simulink model "real_velocity_obs"  (R2023a)
settings: Solver=FixedStepAuto  StartTime=0.0  StopTime=20  FixedStep=0.0005  RelTol=1e-3
undefined symbols (not defined in the file): amp_disp, bias, c, c0, DiscIntNeverNeededParam, dT, freq_disp, k, k0, lsqr_method, m, m0
libraries: fl_lib x14, nesl_utility x8, simulink x3, sharedTrackingLibrary x2
settings Model: Creator=lucabeber  LastModifiedBy=robotics
settings OptimizationCC: ReuseModelBlockBuffer=off

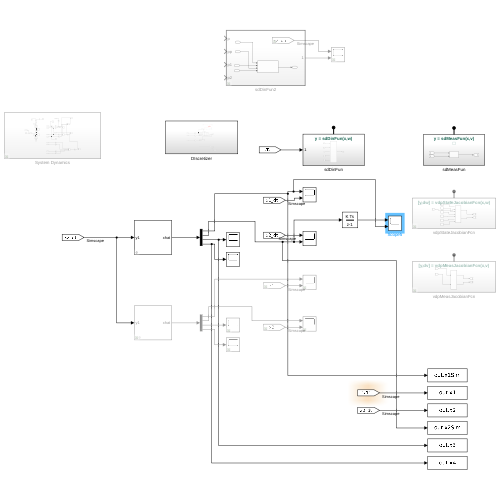
[thumbnail: Simulink's stored preview of the top-level diagram]
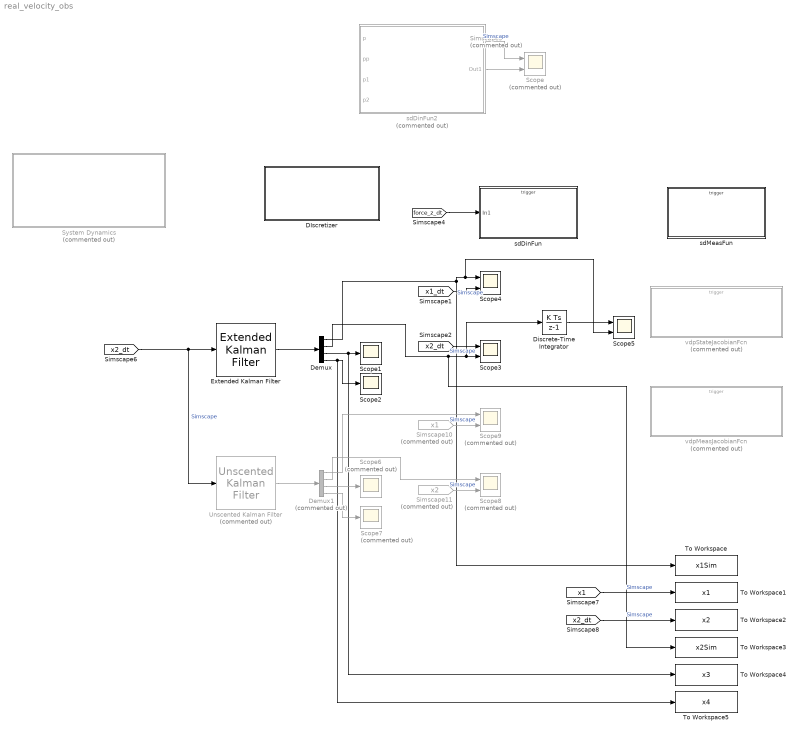
== system real_velocity_obs ==
  DIscretizer : Subsystem
  Demux : Demux
  Demux1 : Demux  Commented=on
  Discrete-Time Integrator : DiscreteIntegrator  SampleTime=-1  ICPrevOutput=DiscIntNeverNeededParam  ICPrevScaledInput=DiscIntNeverNeededParam
  Extended Kalman Filter : sharedTrackingLibrary/Extended Kalman Filter  StateTransitionFcn=sdDinFun  HasStateTransitionJacobianFcn=off  StateTransitionJacobianFcn=vdpStateJacobianFcn  HasAdditiveProcessNoise=Nonadditive  ProcessNoise=1e-5  HasTimeVaryingProcessNoise=off  HasStateTransitionFcnExtraArgument=0  InitialState=[0,0,1000,100]  InitialStateCovariance=[1,1,500,10]  MeasurementFcn1=sdMeasFun  HasMeasurementJacobianFcn1=off  MeasurementJacobianFcn1=vdpMeasJacobianFcn  HasMeasurementEnablePort1=off  HasAdditiveMeasurementNoise1=Nonadditive  MeasurementNoise1=0.000005  HasTimeVaryingMeasurementNoise1=off  HasMeasurementFcnExtraArgument1=0  HasMeasurementWrapping1=off  MeasurementFcn2=myMeasurementFcn  HasMeasurementJacobianFcn2=off  HasMeasurementEnablePort2=off  HasAdditiveMeasurementNoise2=Additive  MeasurementNoise2=1  HasTimeVaryingMeasurementNoise2=off  HasMeasurementFcnExtraArgument2=0  HasMeasurementWrapping2=off  MeasurementFcn3=myMeasurementFcn  HasMeasurementJacobianFcn3=off  HasMeasurementEnablePort3=off  HasAdditiveMeasurementNoise3=Additive  MeasurementNoise3=1  HasTimeVaryingMeasurementNoise3=off  HasMeasurementFcnExtraArgument3=0  HasMeasurementWrapping3=off  MeasurementFcn4=myMeasurementFcn  HasMeasurementJacobianFcn4=off  HasMeasurementEnablePort4=off  HasAdditiveMeasurementNoise4=Additive  MeasurementNoise4=1  HasTimeVaryingMeasurementNoise4=off  HasMeasurementFcnExtraArgument4=0  HasMeasurementWrapping4=off  MeasurementFcn5=myMeasurementFcn  HasMeasurementJacobianFcn5=off  HasMeasurementEnablePort5=off  HasAdditiveMeasurementNoise5=Additive  MeasurementNoise5=1  HasTimeVaryingMeasurementNoise5=off  HasMeasurementFcnExtraArgument5=0  HasMeasurementWrapping5=off  EnableMultirate=off  StateTransitionFcnSampleTime=1  MeasurementFcn1SampleTime=1  MeasurementFcn2SampleTime=1  MeasurementFcn3SampleTime=1  MeasurementFcn4SampleTime=1  MeasurementFcn5SampleTime=1  UseCurrentEstimator=on  OutputStateCovariance=off  DataType=double  SampleTime=dT  NumberOfMeasurements=1
  Scope : Scope  Commented=on  NumInputPorts=2
  Scope1 : Scope
  Scope2 : Scope
  Scope3 : Scope  NumInputPorts=2
  Scope4 : Scope  NumInputPorts=2
  Scope5 : Scope  NumInputPorts=2
  Scope6 : Scope  Commented=on
  Scope7 : Scope  Commented=on
  Scope8 : Scope  Commented=on  NumInputPorts=2
  Scope9 : Scope  Commented=on  NumInputPorts=2
  Simscape10 : From  Commented=on  GotoTag=x1  TagVisibility=global
  Simscape11 : From  Commented=on  GotoTag=x2  TagVisibility=global
  Simscape5 : From  Commented=on  GotoTag=x2_dot  TagVisibility=global
  System Dynamics : Subsystem  Commented=on
  To Workspace : ToWorkspace  VariableName=x1Sim  SampleTime=-1
  To Workspace1 : ToWorkspace  VariableName=x1  SampleTime=-1
  To Workspace2 : ToWorkspace  VariableName=x2  SampleTime=-1
  To Workspace3 : ToWorkspace  VariableName=x2Sim  SampleTime=-1
  To Workspace4 : ToWorkspace  VariableName=x3  SampleTime=-1
  To Workspace5 : ToWorkspace  VariableName=x4  SampleTime=-1
  Unscented Kalman Filter : sharedTrackingLibrary/Unscented Kalman Filter  Commented=on  StateTransitionFcn=sdDinFun  HasAdditiveProcessNoise=Nonadditive  ProcessNoise=0  HasTimeVaryingProcessNoise=off  HasStateTransitionFcnExtraArgument=0  InitialState=[0,0,0,0]  InitialStateCovariance=5000  Alpha=1e-3  Beta=2  Kappa=0  MeasurementFcn1=sdMeasFun  HasMeasurementEnablePort1=off  HasAdditiveMeasurementNoise1=Nonadditive  MeasurementNoise1=0.8  HasTimeVaryingMeasurementNoise1=off  HasMeasurementFcnExtraArgument1=0  HasMeasurementWrapping1=off  MeasurementFcn2=myMeasurementFcn  HasMeasurementEnablePort2=off  HasAdditiveMeasurementNoise2=Additive  MeasurementNoise2=1  HasTimeVaryingMeasurementNoise2=off  HasMeasurementFcnExtraArgument2=0  HasMeasurementWrapping2=off  MeasurementFcn3=myMeasurementFcn  HasMeasurementEnablePort3=off  HasAdditiveMeasurementNoise3=Additive  MeasurementNoise3=1  HasTimeVaryingMeasurementNoise3=off  HasMeasurementFcnExtraArgument3=0  HasMeasurementWrapping3=off  MeasurementFcn4=myMeasurementFcn  HasMeasurementEnablePort4=off  HasAdditiveMeasurementNoise4=Additive  MeasurementNoise4=1  HasTimeVaryingMeasurementNoise4=off  HasMeasurementFcnExtraArgument4=0  HasMeasurementWrapping4=off  MeasurementFcn5=myMeasurementFcn  HasMeasurementEnablePort5=off  HasAdditiveMeasurementNoise5=Additive  MeasurementNoise5=1  HasTimeVaryingMeasurementNoise5=off  HasMeasurementFcnExtraArgument5=0  HasMeasurementWrapping5=off  EnableMultirate=off  StateTransitionFcnSampleTime=1  MeasurementFcn1SampleTime=1  MeasurementFcn2SampleTime=1  MeasurementFcn3SampleTime=1  MeasurementFcn4SampleTime=1  MeasurementFcn5SampleTime=1  UseCurrentEstimator=on  OutputStateCovariance=off  DataType=double  SampleTime=dT  NumberOfMeasurements=1
      settings: LibrarySourceBlock=cstblocks/State Estimation/Unscented Kalman Filter
  sdDinFun : Subsystem  TreatAsAtomicUnit=on
  sdDinFun2 : Subsystem  Commented=on  TreatAsAtomicUnit=on
  sdMeasFun : Subsystem  TreatAsAtomicUnit=on
  vdpMeasJacobianFcn : Subsystem  Commented=on  TreatAsAtomicUnit=on
  vdpStateJacobianFcn : Subsystem  Commented=on  TreatAsAtomicUnit=on
  wires:
  sdDinFun2/1(Out1) -> Scope/2
  Simscape5/1 -> Scope/1  "Simscape"
  [x2_dt] -> Unscented Kalman Filter/1, Extended Kalman Filter/1  "Simscape"
  Extended Kalman Filter/1 -> Demux/1
  Demux/3 -> To Workspace4/1, Scope1/1
  Demux/4 -> To Workspace5/1, Scope2/1
  Demux/1 -> To Workspace/1, Scope5/2, Scope4/1
  Demux/2 -> To Workspace3/1, Discrete-Time Integrator/1, Scope3/2
  [x1_dt] -> Scope4/2  "Simscape"
  [force_z_dt] -> sdDinFun/1(In1)
  Demux1/4 -> Scope7/1
  Demux1/1 -> Scope9/1
  Demux1/3 -> Scope6/1
  Simscape11/1 -> Scope8/2  "Simscape"
  Unscented Kalman Filter/1 -> Demux1/1
  Demux1/2 -> Scope8/1
  Simscape10/1 -> Scope9/2  "Simscape"
  [x2_dt] -> Scope3/1  "Simscape"
  [x1] -> To Workspace1/1  "Simscape"
  [x2_dt] -> To Workspace2/1  "Simscape"
  Discrete-Time Integrator/1 -> Scope5/1

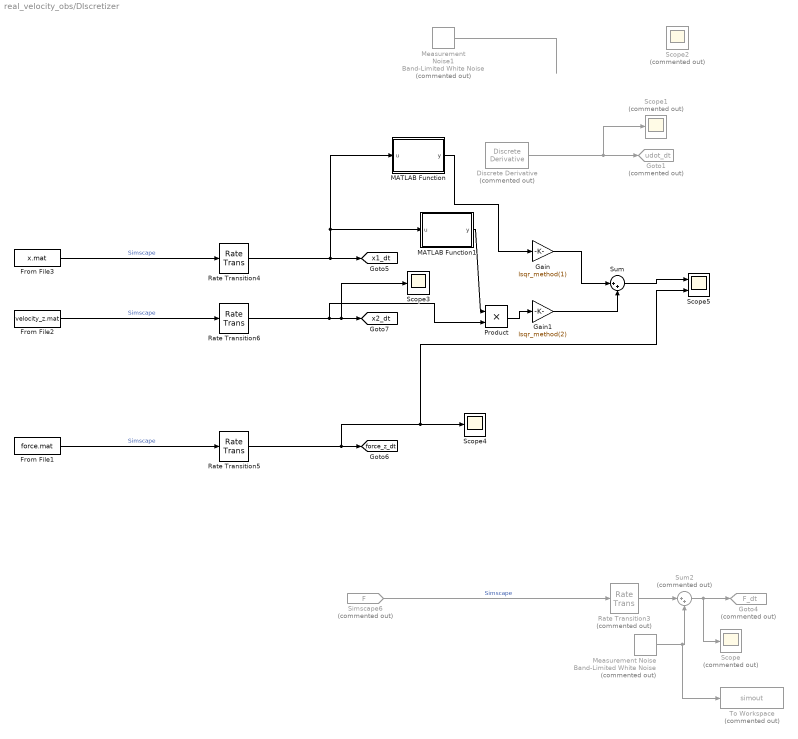
== system real_velocity_obs/DIscretizer ==
  Discrete Derivative : simulink/Discrete/Discrete Derivative  Commented=on  gainval=1.0  ICPrevScaledInput=0.0  OutMin=[]  OutMax=[]  OutDataType=fixdt(1, 16)  OutScaling=2^-10  DoSatur=off
  From File1 : FromFile  FileName=force.mat  SampleTime=dT
  From File2 : FromFile  FileName=velocity_z.mat  SampleTime=dT
  From File3 : FromFile  FileName=x.mat  SampleTime=dT
  Gain : Gain  Gain=lsqr_method(1)
  Gain1 : Gain  Gain=lsqr_method(2)
  Goto1 : Goto  Commented=on  GotoTag=udot_dt  TagVisibility=global
  Goto4 : Goto  Commented=on  GotoTag=F_dt  TagVisibility=global
  MATLAB Function : MATLAB Function  TreatAsAtomicUnit=on
  MATLAB Function1 : MATLAB Function  TreatAsAtomicUnit=on
  Measurement Noise : simulink/Sources/Band-Limited White Noise  Commented=on  Cov=4e-4  Ts=dT  seed=[23342]
  Measurement Noise1 : simulink/Sources/Band-Limited White Noise  Commented=on  Cov=0  Ts=dT  seed=[23342]
  Product : Product
  Rate Transition3 : RateTransition  Commented=on  OutPortSampleTime=dT
  Rate Transition4 : RateTransition  OutPortSampleTime=dT
  Rate Transition5 : RateTransition  OutPortSampleTime=dT
  Rate Transition6 : RateTransition  OutPortSampleTime=dT
  Scope : Scope  Commented=on
  Scope1 : Scope  Commented=on
  Scope2 : Scope  Commented=on
  Scope3 : Scope
  Scope4 : Scope
  Scope5 : Scope  NumInputPorts=2
  Simscape6 : From  Commented=on  GotoTag=F  TagVisibility=global
  Sum : Sum  Inputs=|++
  Sum2 : Sum  Commented=on  Inputs=|++
  To Workspace : ToWorkspace  Commented=on  VariableName=simout  SampleTime=-1
  tag scope: force_z_dt=global, x1_dt=global, x2_dt=global
  wires:
  Simscape6/1 -> Rate Transition3/1  "Simscape"
  Rate Transition3/1 -> Sum2/1
  Sum2/1 -> Scope/1, Goto4/1
  Measurement Noise/1 -> To Workspace/1, Sum2/2
  ? -> Discrete Derivative/1, Scope2/1
  Measurement Noise1/1 -> ?
  Discrete Derivative/1 -> Scope1/1, Goto1/1
  Rate Transition4/1 -> MATLAB Function1/1(u), MATLAB Function/1(u), [x1_dt]
  From File3/1 -> Rate Transition4/1  "Simscape"
  From File2/1 -> Rate Transition6/1  "Simscape"
  Rate Transition6/1 -> Product/2, Scope3/1, [x2_dt]
  From File1/1 -> Rate Transition5/1  "Simscape"
  Rate Transition5/1 -> Scope5/2, Scope4/1, [force_z_dt]
  Sum/1 -> Scope5/1
  Gain/1 -> Sum/1
  Gain1/1 -> Sum/2
  MATLAB Function/1(y) -> Gain/1
  Product/1 -> Gain1/1
  MATLAB Function1/1(y) -> Product/1

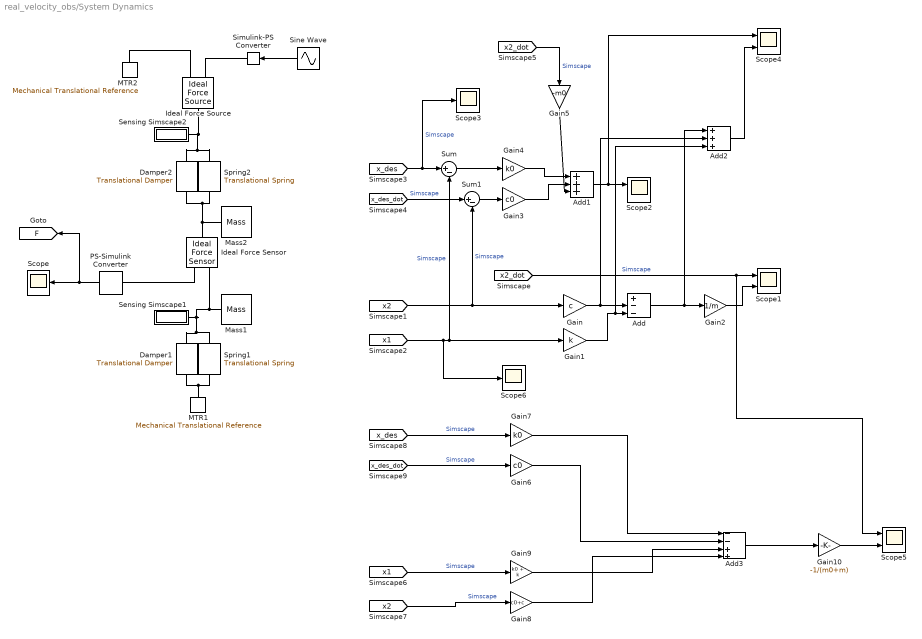
== system real_velocity_obs/System Dynamics ==
  " Spring1" : fl_lib/Mechanical/Translational Elements/Translational Spring  spr_rate=k N/m  v_specify=off  v_priority=None  v=0 m/s  v_nominal_specify=off  v_nominal_unit=m/s  v_nominal_value=1  f_specify=off  f_priority=None  f=0 N  f_nominal_specify=off  f_nominal_unit=N  f_nominal_value=1  x_specify=off  x_priority=High  x=0 m  x_nominal_specify=off  x_nominal_unit=m  x_nominal_value=1
  " Spring2" : fl_lib/Mechanical/Translational Elements/Translational Spring  spr_rate=k0 N/m  v_specify=off  v_priority=None  v=0 m/s  v_nominal_specify=off  v_nominal_unit=m/s  v_nominal_value=1  f_specify=off  f_priority=None  f=0 N  f_nominal_specify=off  f_nominal_unit=N  f_nominal_value=1  x_specify=off  x_priority=High  x=0 m  x_nominal_specify=off  x_nominal_unit=m  x_nominal_value=1
  Add : Sum  Inputs=+--
  Add1 : Sum  Inputs=+++
  Add2 : Sum  Inputs=+++
  Add3 : Sum  Inputs=--++
  Damper1 : fl_lib/Mechanical/Translational Elements/Translational Damper  D=c N/(m/s)  v_specify=off  v_priority=High  v=0 m/s  v_nominal_specify=off  v_nominal_unit=m/s  v_nominal_value=1  f_specify=off  f_priority=High  f=0 N  f_nominal_specify=off  f_nominal_unit=N  f_nominal_value=1
  Damper2 : fl_lib/Mechanical/Translational Elements/Translational Damper  D=c0 N/(m/s)  v_specify=off  v_priority=High  v=0 m/s  v_nominal_specify=off  v_nominal_unit=m/s  v_nominal_value=1  f_specify=off  f_priority=High  f=0 N  f_nominal_specify=off  f_nominal_unit=N  f_nominal_value=1
  Gain : Gain  Gain=c
  Gain1 : Gain  Gain=k
  Gain10 : Gain  Gain=-1/(m0+m)
  Gain2 : Gain  Gain=1/m
  Gain3 : Gain  Gain=c0
  Gain4 : Gain  Gain=k0
  Gain5 : Gain  Gain=-m0
  Gain6 : Gain  Gain=c0
  Gain7 : Gain  Gain=k0
  Gain8 : Gain  Gain=c0+c
  Gain9 : Gain  Gain=k0 + k
  Ideal Force Sensor : fl_lib/Mechanical/Mechanical Sensors/Ideal Force Sensor
  Ideal Force Source : fl_lib/Mechanical/Mechanical Sources/Ideal Force Source
  MTR1 : fl_lib/Mechanical/Translational Elements/Mechanical Translational Reference
  MTR2 : fl_lib/Mechanical/Translational Elements/Mechanical Translational Reference
  Mass1 : fl_lib/Mechanical/Translational Elements/Mass  mass=m kg  num_ports=foundation.enum.numPorts2.one  v_specify=off  v_priority=High  v=0 m/s  v_nominal_specify=off  v_nominal_unit=m/s  v_nominal_value=1  f_specify=off  f_priority=High  f=0 N  f_nominal_specify=off  f_nominal_unit=N  f_nominal_value=1
  Mass2 : fl_lib/Mechanical/Translational Elements/Mass  mass=m0 kg  num_ports=foundation.enum.numPorts2.one  v_specify=off  v_priority=High  v=0 m/s  v_nominal_specify=off  v_nominal_unit=m/s  v_nominal_value=1  f_specify=off  f_priority=High  f=0 N  f_nominal_specify=off  f_nominal_unit=N  f_nominal_value=1
  PS-Simulink Converter : nesl_utility/PS-Simulink Converter  PhysicalDomain=network_engine_domain  SubClassName=ps_output  LeftPortType=input  RightPortType=output  PseudoPeriodic=off  Frequencies=[]  VectorFormat=1-D array  Unit=1  AffineConversion=off
  Scope : Scope
  Scope{1..2,4..5} (4 alike) : Scope  NumInputPorts=2
  Scope3 : Scope
  Scope6 : Scope
  Sensing Simscape1 : Subsystem
      mask Display: disp('v1_sc')
  Sensing Simscape2 : Subsystem
      mask Display: disp('v2_sc')
  Simulink-PS Converter : nesl_utility/Simulink-PS Converter  PhysicalDomain=network_engine_domain  SubClassName=ps_input  LeftPortType=input  RightPortType=output  PseudoPeriodic=off  Frequencies=[]  NoiseDistribution=none  NoiseParameters=[]  Unit=1  AffineConversion=off  FilteringAndDerivatives=provide  SimscapeFilterOrder=1  InputFilterTimeConstant=0.001  UdotUserProvided=0
  Sine Wave : Sin  Amplitude=amp_disp  Bias=bias  Frequency=freq_disp*2*pi  SampleTime=0
  Sum : Sum  Inputs=|+-
  Sum1 : Sum  Inputs=|+-
  tag scope: F=global
  wires:
  [x_des_dot] -> Sum1/1  "Simscape"
  Gain/1 -> Add2/2, Add/2
  Sum1/1 -> Gain3/1
  Add/1 -> Add2/1, Gain2/1
  Gain3/1 -> Add1/2
  Gain2/1 -> Scope1/2
  Gain4/1 -> Add1/1
  PS-Simulink Converter/1 -> [F], Scope/1
  [x2] -> Gain/1, Sum1/2  "Simscape"
  [x_des] -> Scope3/1, Sum/1  "Simscape"
  [x1] -> Scope6/1, Sum/2, Gain1/1  "Simscape"
  Sum/1 -> Gain4/1
  Gain1/1 -> Add2/3, Add/3
  Sine Wave/1 -> Simulink-PS Converter/1
  Gain5/1 -> Add1/3
  [x2_dot] -> Gain5/1  "Simscape"
  [x2_dot] -> Scope5/1, Scope1/1  "Simscape"
  Add1/1 -> Scope4/1, Scope2/1
  Add2/1 -> Scope4/2
  [x_des] -> Gain7/1  "Simscape"
  Gain7/1 -> Add3/1
  [x_des_dot] -> Gain6/1  "Simscape"
  Gain6/1 -> Add3/2
  [x1] -> Gain9/1  "Simscape"
  [x2] -> Gain8/1  "Simscape"
  Gain9/1 -> Add3/3
  Gain8/1 -> Add3/4
  Add3/1 -> Gain10/1
  Gain10/1 -> Scope5/2
  connections:
  Ideal Force Source/RConn1 -- Simulink-PS Converter/RConn1
  Ideal Force Source/RConn2 -- MTR2/LConn1
  PS-Simulink Converter/LConn1 -- Ideal Force Sensor/RConn2
  MTR1/LConn1 -- " Spring1"/RConn1 -- Damper1/RConn1
  Mass2/LConn1 -- " Spring2"/RConn1 -- Damper2/RConn1 -- Ideal Force Sensor/LConn1
  Damper2/LConn1 -- " Spring2"/LConn1 -- Ideal Force Source/LConn1 -- Sensing Simscape2/LConn1
  Damper1/LConn1 -- " Spring1"/LConn1 -- Sensing Simscape1/LConn1 -- Ideal Force Sensor/RConn1 -- Mass1/LConn1

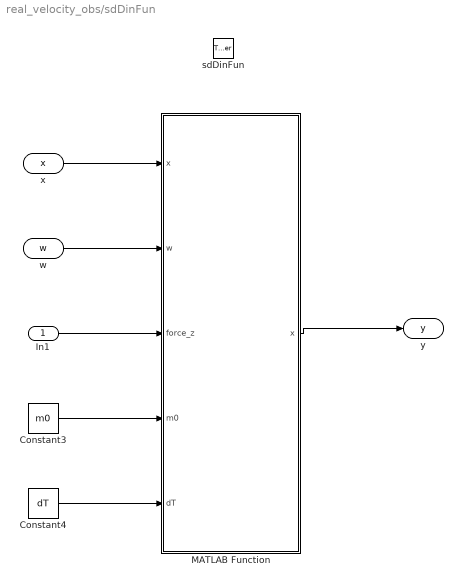
== system real_velocity_obs/sdDinFun ==
  In1 : Inport
  sdDinFun : TriggerPort  TriggerType=function-call  IsSimulinkFunction=on  FunctionName=sdDinFun  FunctionVisibility=scoped  VariantControl=(inherit)
  Constant3 : Constant  Value=m0
  Constant4 : Constant  Value=dT
  MATLAB Function : MATLAB Function  TreatAsAtomicUnit=on
  x : ArgIn  DisableCoverage=on  PortDimensions=4  ArgumentName=x
  w : ArgIn  DisableCoverage=on  Port=2  ArgumentName=w
  y : ArgOut  DisableCoverage=on  PortDimensions=4  ArgumentName=y
  wires:
  MATLAB Function/1(x) -> y/1
  x/1 -> MATLAB Function/1("x ")
  w/1 -> MATLAB Function/2(w)
  In1/1 -> MATLAB Function/3(force_z)
  Constant4/1 -> MATLAB Function/5(dT)
  Constant3/1 -> MATLAB Function/4(m0)

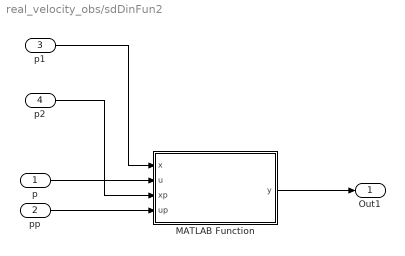
== system real_velocity_obs/sdDinFun2 ==
  p : Inport
  pp : Inport  Port=2
  p1 : Inport  Port=3
  p2 : Inport  Port=4
  MATLAB Function : MATLAB Function  TreatAsAtomicUnit=on
  Out1 : Outport
  wires:
  MATLAB Function/1(y) -> Out1/1
  p1/1 -> MATLAB Function/1(x)
  p2/1 -> MATLAB Function/3(xp)
  pp/1 -> MATLAB Function/4(up)
  p/1 -> MATLAB Function/2(u)

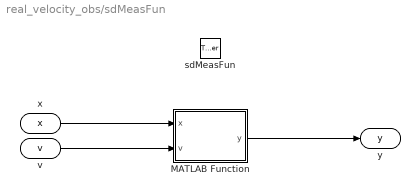
== system real_velocity_obs/sdMeasFun ==
  sdMeasFun : TriggerPort  TriggerType=function-call  IsSimulinkFunction=on  FunctionName=sdMeasFun  FunctionVisibility=scoped  VariantControl=(inherit)
  MATLAB Function : MATLAB Function  TreatAsAtomicUnit=on
  x : ArgIn  DisableCoverage=on  PortDimensions=4  ArgumentName=x
  v : ArgIn  DisableCoverage=on  Port=2  ArgumentName=v
  y : ArgOut  DisableCoverage=on  ArgumentName=y
  wires:
  MATLAB Function/1(y) -> y/1
  x/1 -> MATLAB Function/1(x)
  v/1 -> MATLAB Function/2(v)

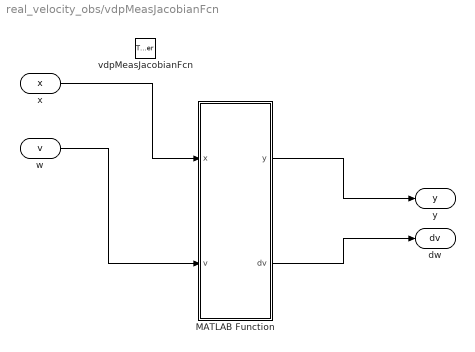
== system real_velocity_obs/vdpMeasJacobianFcn ==
  vdpMeasJacobianFcn : TriggerPort  TriggerType=function-call  IsSimulinkFunction=on  FunctionName=vdpMeasJacobianFcn  FunctionVisibility=scoped  VariantControl=(inherit)
  MATLAB Function : MATLAB Function  TreatAsAtomicUnit=on
  x : ArgIn  DisableCoverage=on  PortDimensions=4  ArgumentName=x
  w : ArgIn  DisableCoverage=on  Port=2  ArgumentName=v
  y : ArgOut  DisableCoverage=on  PortDimensions=[1,4]  ArgumentName=y
  dw : ArgOut  DisableCoverage=on  Port=2  ArgumentName=dv
  wires:
  MATLAB Function/1(y) -> y/1
  x/1 -> MATLAB Function/1(x)
  w/1 -> MATLAB Function/2(v)
  MATLAB Function/2(dv) -> dw/1

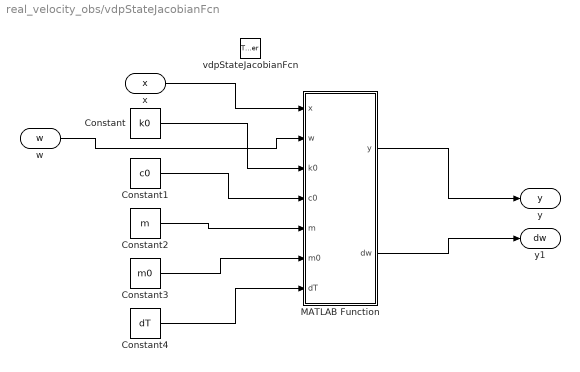
== system real_velocity_obs/vdpStateJacobianFcn ==
  vdpStateJacobianFcn : TriggerPort  TriggerType=function-call  IsSimulinkFunction=on  FunctionName=vdpStateJacobianFcn  FunctionVisibility=scoped  VariantControl=(inherit)
  Constant : Constant  Value=k0
  Constant1 : Constant  Value=c0
  Constant2 : Constant  Value=m
  Constant3 : Constant  Value=m0
  Constant4 : Constant  Value=dT
  MATLAB Function : MATLAB Function  TreatAsAtomicUnit=on
  x : ArgIn  DisableCoverage=on  PortDimensions=4  ArgumentName=x
  w : ArgIn  DisableCoverage=on  Port=2  ArgumentName=w
  y : ArgOut  DisableCoverage=on  PortDimensions=[4,4]  ArgumentName=y
  y1 : ArgOut  DisableCoverage=on  Port=2  PortDimensions=4  ArgumentName=dw
  wires:
  MATLAB Function/1(y) -> y/1
  x/1 -> MATLAB Function/1(x)
  Constant1/1 -> MATLAB Function/4(c0)
  Constant3/1 -> MATLAB Function/6(m0)
  Constant4/1 -> MATLAB Function/7(dT)
  Constant/1 -> MATLAB Function/3(k0)
  Constant2/1 -> MATLAB Function/5(m)
  w/1 -> MATLAB Function/2(w)
  MATLAB Function/2(dw) -> y1/1

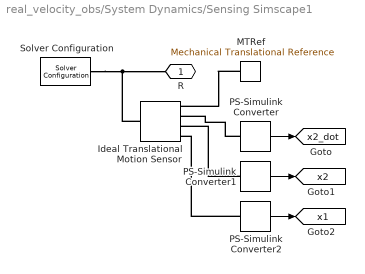
== system real_velocity_obs/System Dynamics/Sensing Simscape1 ==
  Ideal Translational Motion Sensor : fl_lib/Mechanical/Mechanical Sensors/Ideal Translational Motion Sensor  reference=foundation.enum.MeasurementReference.difference  acceleration_port=true  velocity_port=true  position_port=true  offset=0 m
      settings: InternalSimscapePortConfiguration="{\"Bottom\":[],\"Left\":[{\"id\":\"R\",\"label\":\"R\",\"type\":\"foundation.mechanical.translational.translational\"}],\"Right\":[{\"id\":\"C\",\"label\":\"C\",\"type\":\"foundation.mechanical.translational.translational\"},{\"id\":\"A\",\"label\":\"A\",\"type\":\"output\"},{\"id\":\"V\",\"label\":\"V\",\"type\":\"output\"},{\"id\":\"P\",\"label\":\"P\",\"type\":\"output\"}],\"Top\":[]}"
  MTRef : fl_lib/Mechanical/Translational Elements/Mechanical Translational Reference
  PS-Simulink Converter : nesl_utility/PS-Simulink Converter  PhysicalDomain=network_engine_domain  SubClassName=ps_output  LeftPortType=input  RightPortType=output  PseudoPeriodic=off  Frequencies=[]  VectorFormat=1-D array  Unit=1  AffineConversion=off
  PS-Simulink Converter1 : nesl_utility/PS-Simulink Converter  PhysicalDomain=network_engine_domain  SubClassName=ps_output  LeftPortType=input  RightPortType=output  PseudoPeriodic=off  Frequencies=[]  VectorFormat=1-D array  Unit=1  AffineConversion=off
  PS-Simulink Converter2 : nesl_utility/PS-Simulink Converter  PhysicalDomain=network_engine_domain  SubClassName=ps_output  LeftPortType=input  RightPortType=output  PseudoPeriodic=off  Frequencies=[]  VectorFormat=1-D array  Unit=1  AffineConversion=off
  Solver Configuration : nesl_utility/Solver Configuration  PhysicalDomain=network_engine_domain  SubClassName=solver  LeftPortType=input  RightPortType=generic  Tones=[]  Harmonics=[]  SimulateNoise=off  Profile=off  UseLocalSampling=off  EnableSwitchedLinearOptims=on  FrequencyDomain=off  UseCCode=off  RelTol=0.001  AbsTol=1e-06  MinStep=1e-09  ToWorkspace=off  RevertToSquareIcSolve=off  NumHomotopyIterations=100  PhasorMode=off  PhasorModeNumHarmonics=1  ConsistencySolver=NEWTON_XTOL_AFTER_FTOL  IndexReductionMethod=DerivativeReplacement  DoDC=off  ResidualTolerance=1e-9  ConsistencyTolSource=GLOBAL  ConsistencyAbsTol=0.001  ConsistencyRelTol=0.001  ConsistencyTolFactor=0.001  UseLocalSolver=off  LocalSolverChoice=NE_BACKWARD_EULER_ADVANCER  ResolveIndetEquations=on  FunctionEvalNumThread=1  LocalSolverSampleTime=.001  DoFixedCost=off  MaxNonlinIter=12  MaxModeIter=2  ComputeImpulses=off  ImpulseIterations=2  LinearAlgebra=auto  LinearAlgebraNumThread=0  EquationFormulation=NE_TIME_EF  DelaysMemoryBudget=1024  AutomaticFiltering=on  FilteringTimeConstant=0.001  PartitionStorageMethod=AS_NEEDED  PartitionMemoryBudget=1024  PartitionMethod=FAST
  R : PMIOPort  Side=Left
  tag scope: x1=global, x2=global, x2_dot=global
  wires:
  PS-Simulink Converter/1 -> [x2_dot]
  PS-Simulink Converter1/1 -> [x2]
  PS-Simulink Converter2/1 -> [x1]
  connections:
  MTRef/LConn1 -- Ideal Translational Motion Sensor/RConn1
  Ideal Translational Motion Sensor/LConn1 -- Solver Configuration/RConn1 -- R/RConn1
  PS-Simulink Converter2/LConn1 -- Ideal Translational Motion Sensor/RConn4
  PS-Simulink Converter1/LConn1 -- Ideal Translational Motion Sensor/RConn3
  PS-Simulink Converter/LConn1 -- Ideal Translational Motion Sensor/RConn2

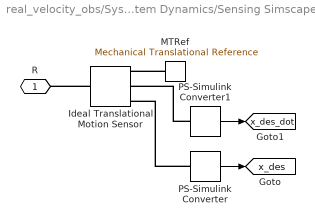
== system real_velocity_obs/System Dynamics/Sensing Simscape2 ==
  Ideal Translational Motion Sensor : fl_lib/Mechanical/Mechanical Sensors/Ideal Translational Motion Sensor  reference=foundation.enum.MeasurementReference.difference  acceleration_port=false  velocity_port=true  position_port=true  offset=0 m
  MTRef : fl_lib/Mechanical/Translational Elements/Mechanical Translational Reference
  PS-Simulink Converter : nesl_utility/PS-Simulink Converter  PhysicalDomain=network_engine_domain  SubClassName=ps_output  LeftPortType=input  RightPortType=output  PseudoPeriodic=off  Frequencies=[]  VectorFormat=1-D array  Unit=1  AffineConversion=off
  PS-Simulink Converter1 : nesl_utility/PS-Simulink Converter  PhysicalDomain=network_engine_domain  SubClassName=ps_output  LeftPortType=input  RightPortType=output  PseudoPeriodic=off  Frequencies=[]  VectorFormat=1-D array  Unit=1  AffineConversion=off
  R : PMIOPort  Side=Left
  tag scope: x_des=global, x_des_dot=global
  wires:
  PS-Simulink Converter/1 -> [x_des]
  PS-Simulink Converter1/1 -> [x_des_dot]
  connections:
  Ideal Translational Motion Sensor/LConn1 -- R/RConn1
  PS-Simulink Converter/LConn1 -- Ideal Translational Motion Sensor/RConn3
  MTRef/LConn1 -- Ideal Translational Motion Sensor/RConn1
  PS-Simulink Converter1/LConn1 -- Ideal Translational Motion Sensor/RConn2

== matlab function real_velocity_obs/sdDinFun/MATLAB Function ==
  data: x input; x output; w input; force_z input; m0 input; dT input
function x = sdDinFun(x,w,force_z,m0,dT)
  

% stiffness contribution
%sc = -  4/3 * (4 * x(3)) * x(1) * sqrt(2*R1*x(1));
%sc = -x(1)*x(3);
% damping constribution
%dc = - 2 * (4*x(4)) * sqrt(2*R1*x(1)) * x(2);
%dc = -x(2)*x(4);

x = [
    x(1) + dT * x(2);
    x(2) + dT/(m0)*( force_z - abs(x(1))^(1.35) * x(3) -  x(2) * x(4) * abs(x(1))^(0.45) ) + w;
    x(3);
    x(4); 
];
% 
% x = [
%     x(1) + dT * x(2);
%     x(2) + (dT/m)*( k0*(u - x(1)) + c0*(ud - x(2)) -  4/3 * (4 * x(3)) * x(1) * sqrt(abs(2*R1*x(1))) ...
%     - 2 * (4*x(4)) * sqrt(abs(2*R1*x(1))) * x(2)) + w;
%     x(3);
%     x(4); 
% ];

== matlab function real_velocity_obs/sdMeasFun/MATLAB Function ==
  data: x input; y output; v input
function y = fnc(x,v)

y = abs(x(1))^(1.35)*x(3) + x(2)*x(4)*abs(x(1))^(0.45) + v;
%y = x(2) + v;
end

== matlab function real_velocity_obs/sdDinFun2/MATLAB Function ==
  data: x input; u input; y output; xp input; up input
function y = fnc(x,u,xp,up)
dT = 1/(2e3); % s
m = 1; % kg
amp_disp = 0.01; % m
freq_disp = 5; % Hz
k0 = 1500; % N/m
c0 = 40; % N/(m/s)
k = 1000; % N
c = 20; % N/(m/s) 
   

% stiffness contribution
%sc = -  4/3 * (4 * x(3)) * x(1) * sqrt(2*R1*x(1));
%sc = -x(1)*x(3);
% damping constribution
%dc = - 2 * (4*x(4)) * sqrt(2*R1*x(1)) * x(2);
%dc = -x(2)*x(4);

y = 1/m*(k0*(u - x) + c0*(up - xp) - x*k - xp*c);

== matlab function real_velocity_obs/vdpStateJacobianFcn/MATLAB Function ==
  data: x input; w input; y output; k0 input; c0 input; m input; m0 input; dT input; dw output
function [y,dw] = fnc(x,w,k0,c0,m,m0,dT)

y = [
    1, dT, 0, 0;
    -(dT * (x(3) + k0)) / (m + m0), 1 - (dT * (x(4) + c0)) / (m + m0), -(dT * x(1)) / (m + m0), -(dT * x(2) )/ (m + m0);
    0, 0, 1, 0;
    0, 0, 0, 1
];

dw = [
    0,1,0,0
];

end

== matlab function real_velocity_obs/vdpMeasJacobianFcn/MATLAB Function ==
  data: x input; v input; y output; dv output
function [y,dv] = fnc(x,v)

y = [
    0,1,0,0
];

dv = [
    1
];

end

== matlab function real_velocity_obs/DIscretizer/MATLAB Function ==
  data: u input; y output
function y = fcn(u)

y = abs(u)^(1.35);

== matlab function real_velocity_obs/DIscretizer/MATLAB Function1 ==
  data: u input; y output
function y = fcn(u)

y = abs(u)^(0.45);
